simulink model "exampleVapourPressure"  (Simulink 7.6)
settings: Solver=ode45  StartTime=0.0  StopTime=10.0  RelTol=1e-3
libraries: carnot x4
settings Model: Creator=drhf  LastModifiedBy=drhf

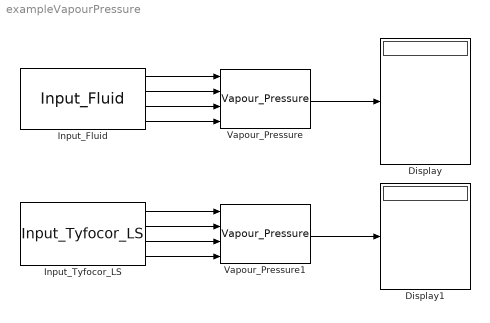
== system exampleVapourPressure ==
  Display : Display
  Display1 : Display
  Input_Fluid : carnot/Basic/Material_Properties/Input_Fluid  SystemSampleTime=-1  fluid=water  T=[0:20:100]  p=1013e2  x=0.005
  Input_Tyfocor_LS : carnot/Basic/Material_Properties/Input_Tyfocor_LS  SystemSampleTime=-1  T=10:20:90  p=1e5
  Vapour_Pressure : carnot/Basic/Material_Properties/Vapour_Pressure  SystemSampleTime=-1
  Vapour_Pressure1 : carnot/Basic/Material_Properties/Vapour_Pressure  SystemSampleTime=-1
  wires:
  Input_Fluid/1 -> Vapour_Pressure/1
  Input_Fluid/2 -> Vapour_Pressure/2
  Input_Fluid/3 -> Vapour_Pressure/3
  Input_Fluid/4 -> Vapour_Pressure/4
  Vapour_Pressure/1 -> Display/1
  Input_Tyfocor_LS/1 -> Vapour_Pressure1/1
  Input_Tyfocor_LS/2 -> Vapour_Pressure1/2
  Input_Tyfocor_LS/3 -> Vapour_Pressure1/3
  Input_Tyfocor_LS/4 -> Vapour_Pressure1/4
  Vapour_Pressure1/1 -> Display1/1
